simulink model "VehicleSystemControl"  (R2023a)
settings: Solver=VariableStepAuto  StartTime=0.0  StopTime=4  RelTol=1e-3
PreLoadFcn:
  | J = 0.22619921148445760000;
  | c = 8.89069171842483820000;
  | k = 19.15595408068224300000;
  | input_delay = 0.00986306560803374390;
  | 
  | Kt = 174.53000000000000000000;
  | angle_init = 15.00000000000000000000;
  | angle_open = 90.00000000000000000000;
  | Ts = 0.005;
undefined symbols (not defined in the file): units
libraries: simulink x1
CloseFcn:
  | clear J c k input_delay Kt angle_init angle_open Ts
Description:
  | Throttle Position Control System Model
  | This model represents the throttle position control system controlling a throttle body
settings Model: Creator=The MathWorks, Inc.  LastModifiedBy=omert
settings SolverCC: AlgebraicLoopSolver=TrustRegion
settings DebuggingCC: IntegerOverflowMsg=error  UnconnectedInputMsg=warning  UnconnectedOutputMsg=warning  UnconnectedLineMsg=warning  SFExecutionAtInitializationDiag=none
settings RTWCC: DLArmComputeVersion=19.05

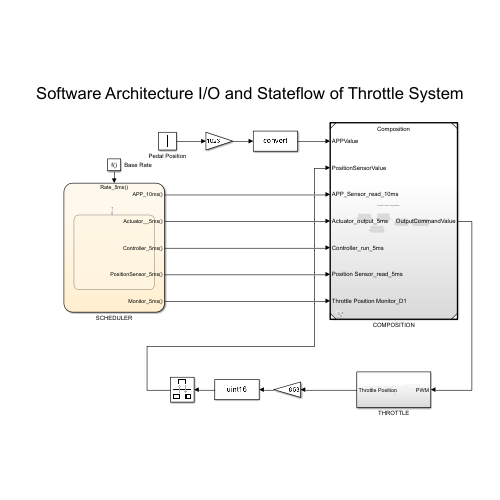
[thumbnail: Simulink's stored preview of the top-level diagram]
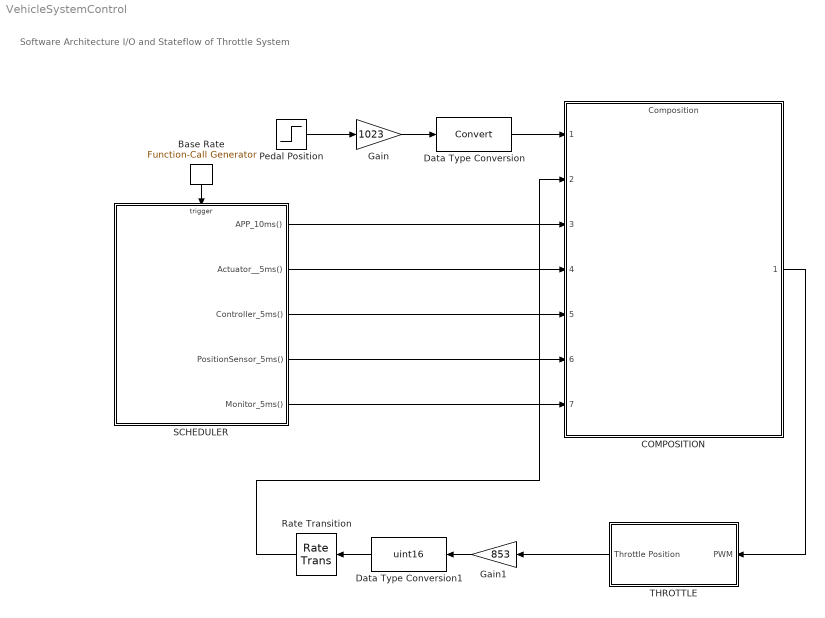
== system VehicleSystemControl ==
  note: Software Architecture I/O and Stateflow of Throttle System
  Base Rate : simulink/Ports & Subsystems/Function-Call Generator  sample_time=0.05  numberOfIterations=1  DisallowWideOutput=off
  COMPOSITION : ModelReference  ModelNameDialog=Composition  SimulationMode=Normal  ScheduleRates=on  ModelReferenceVersion=5.7
  Data Type Conversion : DataTypeConversion  SaturateOnIntegerOverflow=off  RndMeth=Floor
  Data Type Conversion1 : DataTypeConversion  OutDataTypeStr=uint16  SaturateOnIntegerOverflow=off  RndMeth=Floor
  Gain : Gain  Gain=1023
  Gain1 : Gain  Gain=853
  Pedal Position : Step  Time=0.25  SampleTime=0.05
  Rate Transition : RateTransition
  SCHEDULER : Stateflow chart  TreatAsAtomicUnit=on
  THROTTLE : Subsystem
  wires:
  SCHEDULER/1(APP_10ms()) -> COMPOSITION/3
  SCHEDULER/5(Monitor_5ms()) -> COMPOSITION/7
  SCHEDULER/2(Actuator__5ms()) -> COMPOSITION/4
  SCHEDULER/3(Controller_5ms()) -> COMPOSITION/5
  SCHEDULER/4(PositionSensor_5ms()) -> COMPOSITION/6
  Data Type Conversion/1 -> COMPOSITION/1
  Base Rate/1 -> SCHEDULER/Trigger
  Gain/1 -> Data Type Conversion/1
  Pedal Position/1 -> Gain/1
  COMPOSITION/1 -> THROTTLE/1(PWM)
  Gain1/1 -> Data Type Conversion1/1
  Data Type Conversion1/1 -> Rate Transition/1
  THROTTLE/1(Throttle Position) -> Gain1/1
  Rate Transition/1 -> COMPOSITION/2

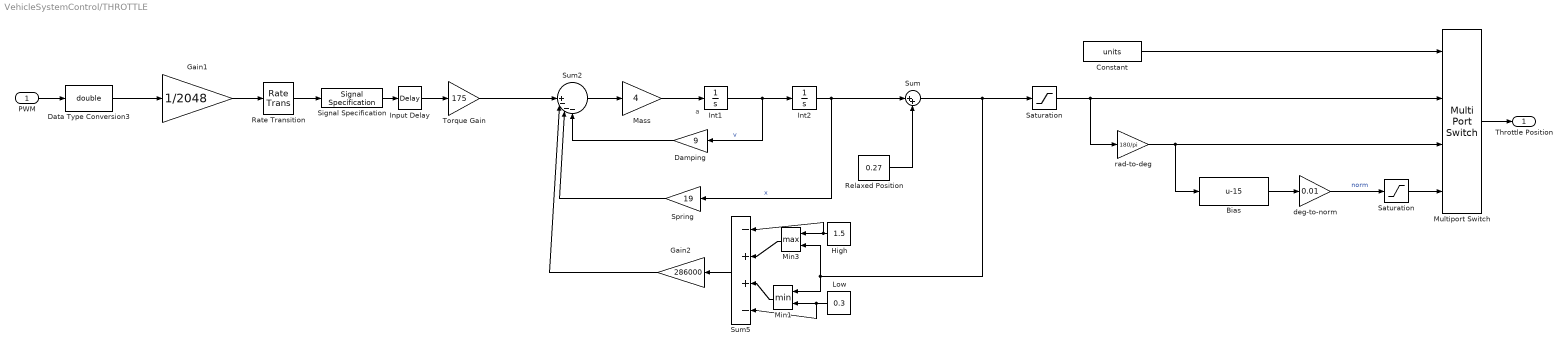
== system VehicleSystemControl/THROTTLE ==
  note: a
  PWM : Inport
  Bias : Bias  Bias=-15  SaturateOnIntegerOverflow=off
  Constant : Constant  Value=units
  Damping : Gain  Gain=9  SaturateOnIntegerOverflow=on  OutDataTypeStr=Inherit: Same as input  ParamDataTypeStr=Inherit: Same as input
  Data Type Conversion3 : DataTypeConversion  OutDataTypeStr=double  SaturateOnIntegerOverflow=off  RndMeth=Floor
  Gain1 : Gain  Gain=1/2048
  Gain2 : Gain  Gain=286000  SaturateOnIntegerOverflow=on  OutDataTypeStr=Inherit: Same as input  ParamDataTypeStr=Inherit: Same as input
  High : Constant  Value=1.5
  Input Delay : TransportDelay  DelayTime=0.01  FixedBuffer=on
  Int1 : Integrator
  Int2 : Integrator
  Low : Constant  Value=0.3
  Mass : Gain  Gain=4  SaturateOnIntegerOverflow=on  OutDataTypeStr=Inherit: Same as input  ParamDataTypeStr=Inherit: Same as input
  Min1 : MinMax  Inputs=2  InputSameDT=on  SaturateOnIntegerOverflow=on
  Min3 : MinMax  Function=max  Inputs=2  InputSameDT=on  SaturateOnIntegerOverflow=on
  Multiport Switch : MultiPortSwitch  SaturateOnIntegerOverflow=off  InputSameDT=off
  Rate Transition : RateTransition
  Relaxed Position : Constant  Value=0.27
  Saturation : Saturate  UpperLimit=pi/2  LowerLimit=0.0
  "Saturation " : Saturate  UpperLimit=1.0  LowerLimit=0.0
  Signal Specification : SignalSpecification  SampleTime=0
  Spring : Gain  Gain=19  SaturateOnIntegerOverflow=on  OutDataTypeStr=Inherit: Same as input  ParamDataTypeStr=Inherit: Same as input
  Sum : Sum  Inputs=|++  InputSameDT=on  SaturateOnIntegerOverflow=on  OutDataTypeStr=Inherit: Same as first input
  Sum2 : Sum  Inputs=|||+---  InputSameDT=on  SaturateOnIntegerOverflow=on  OutDataTypeStr=Inherit: Same as first input
  Sum5 : Sum  Inputs=-+||+-  InputSameDT=on  SaturateOnIntegerOverflow=on  OutDataTypeStr=Inherit: Same as first input
  Torque Gain : Gain  Gain=175  SaturateOnIntegerOverflow=on  OutDataTypeStr=Inherit: Same as input  ParamDataTypeStr=Inherit: Same as input
  deg-to-norm : Gain  Gain=0.01
      settings: AttributesFormatString=%<Gain>
  rad-to-deg : Gain  Gain=180/pi
  Throttle Position : Outport  VectorParamsAs1DForOutWhenUnconnected=off
  wires:
  Damping/1 -> Sum2/4
  Sum/1 -> Min3/2, Min1/1, Saturation/1
  "Saturation "/1 -> Multiport Switch/4
  Gain1/1 -> Rate Transition/1
  Saturation/1 -> rad-to-deg/1, Multiport Switch/2
  deg-to-norm/1 -> "Saturation "/1  "norm"
  rad-to-deg/1 -> Multiport Switch/3, Bias/1
  Sum5/1 -> Gain2/1
  Constant/1 -> Multiport Switch/1
  Gain2/1 -> Sum2/2
  Bias/1 -> deg-to-norm/1
  Signal Specification/1 -> Input Delay/1
  Sum2/1 -> Mass/1
  High/1 -> Sum5/1, Min3/1
  Low/1 -> Min1/2, Sum5/4
  Int2/1 -> Spring/1, Sum/1  "x"
  Int1/1 -> Damping/1, Int2/1  "v"
  Input Delay/1 -> Torque Gain/1
  Data Type Conversion3/1 -> Gain1/1
  Relaxed Position/1 -> Sum/2
  Spring/1 -> Sum2/3
  Mass/1 -> Int1/1
  Multiport Switch/1 -> Throttle Position/1
  Min1/1 -> Sum5/3
  Rate Transition/1 -> Signal Specification/1
  PWM/1 -> Data Type Conversion3/1
  Min3/1 -> Sum5/2
  Torque Gain/1 -> Sum2/1

== stateflow chart VehicleSystemControl/SCHEDULER ==
  state Run
    en:
    TPS_Primary_read_5ms();
    TP_Monitor_select_5ms();
    Controller_run_5ms();
    Actuator_output_5ms();
    APP_read_10ms();
    on every(1, base_rate_5ms):
    TPS_Primary_read_5ms();
    TP_Monitor_select_5ms();
    Controller_run_5ms();
    Actuator_output_5ms();
    on every(2, base_rate_5ms):
    APP_read_10ms();
  (default) -> Run
  events: APP_10ms output FUNCTION_CALL_EVENT; Actuator__5ms output FUNCTION_CALL_EVENT; Controller_5ms output FUNCTION_CALL_EVENT; PositionSensor_5ms output FUNCTION_CALL_EVENT; Monitor_5ms output FUNCTION_CALL_EVENT; Rate_5ms input FUNCTION_CALL_EVENT
